simulink model "linearized_wave_model"  (R2020a)
settings: Solver=FixedStepAuto  StartTime=0.0  StopTime=2000  RelTol=1e-3
values from neighbouring files (symbols this model uses):
  east_drift_limit = 2    [wave_parameters.mat]
  k_down = 1.3    [wave_parameters.mat]
  k_east = 2    [wave_parameters.mat]
  k_north = 2    [wave_parameters.mat]
  k_pitch = 3    [wave_parameters.mat]
  k_roll = 3    [wave_parameters.mat]
  k_yaw = 3    [wave_parameters.mat]
  north_drift_limit = 2    [wave_parameters.mat]
  peak_frequency = 0.8    [wave_parameters.mat]
  wave_height = 1    [wave_parameters.mat]
  yaw_drift_limit = 0.174532925199    [wave_parameters.mat]
libraries: simulink x9
settings Model: Creator=thomas.evang  LastModifiedBy=thomas.evang
settings RTWCC: Description=Generic Real-Time Target

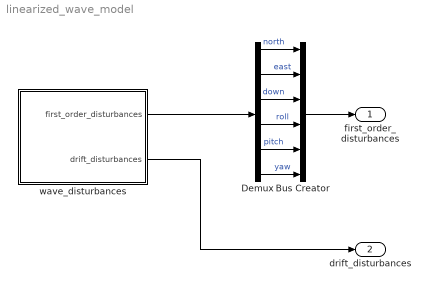
== system linearized_wave_model ==
  Bus Creator : BusCreator  Inputs=6  OutDataTypeStr=Bus: wave_disturbance
  Demux : Demux  Outputs=6
  wave_disturbances : Subsystem  mask{Hs=wave_height, w0=peak_frequency, k_north=k_north, k_east=k_east, k_down=k_down, k_roll=k_roll, k_pitch=k_pitch, k_yaw=k_yaw}
      mask prompts: Hs "Significant Wave Height"; w0 "Peak Frequency"; k_north "North Coefficient"; k_east "East Coefficient"; k_down "Down Coefficient"; k_roll "Roll Coefficient"; k_pitch "Pitch Coefficient"; k_yaw "Yaw Coefficient"
  first_order_disturbances : Outport  OutDataTypeStr=Bus: wave_disturbance
  drift_disturbances : Outport  Port=2  OutDataTypeStr=Bus: position_6dof
  wires:
  wave_disturbances/1(first_order_disturbances) -> Demux/1
  Demux/2 -> Bus Creator/2  "east"
  Demux/1 -> Bus Creator/1  "north"
  Demux/3 -> Bus Creator/3  "down"
  Demux/4 -> Bus Creator/4  "roll"
  Demux/5 -> Bus Creator/5  "pitch"
  Demux/6 -> Bus Creator/6  "yaw"
  Bus Creator/1 -> first_order_disturbances/1
  wave_disturbances/2(drift_disturbances) -> drift_disturbances/1

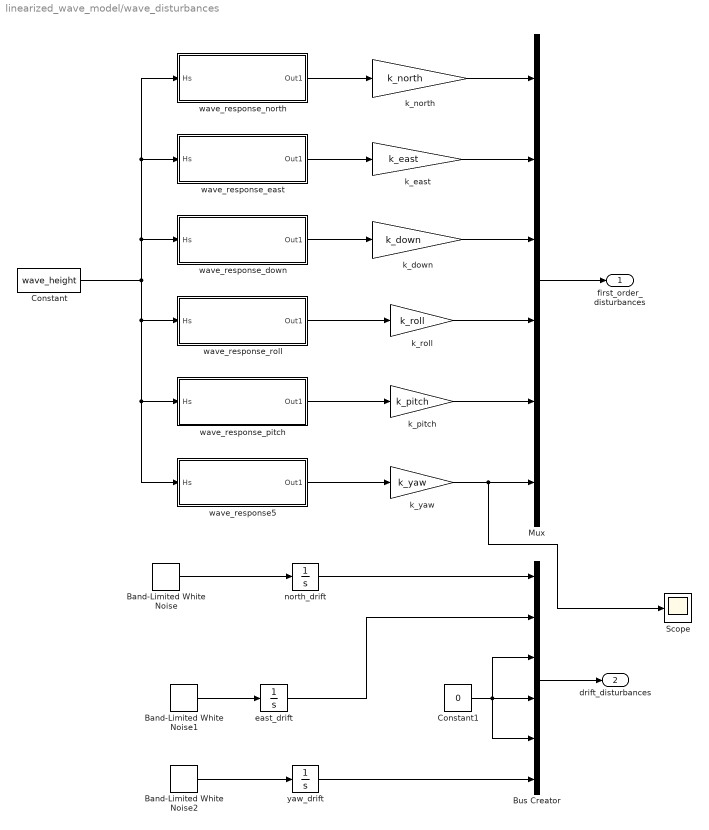
== system linearized_wave_model/wave_disturbances ==
  Band-Limited White Noise : simulink/Sources/Band-Limited White Noise  Cov=[0.005]  Ts=0.1  seed=[23341]
  Band-Limited White Noise1 : simulink/Sources/Band-Limited White Noise  Cov=[0.005]  Ts=0.1  seed=[23341]
  Band-Limited White Noise2 : simulink/Sources/Band-Limited White Noise  Cov=[0.005]  Ts=0.1  seed=[23341]
  Bus Creator : BusCreator  Inputs=6  OutDataTypeStr=Bus: position_6dof
      settings: InheritFromInputs=off
  Constant : Constant  Value=wave_height
  Constant1 : Constant  Value=0
  Mux : Mux  Inputs=6
  Scope : Scope
  east_drift : Integrator  LimitOutput=on  UpperSaturationLimit=east_drift_limit  LowerSaturationLimit=-east_drift_limit
  k_down : Gain  Gain=k_down
  k_east : Gain  Gain=k_east
  k_north : Gain  Gain=k_north
  k_pitch : Gain  Gain=k_pitch
  k_roll : Gain  Gain=k_roll
  k_yaw : Gain  Gain=k_yaw
  north_drift : Integrator  LimitOutput=on  UpperSaturationLimit=north_drift_limit  LowerSaturationLimit=-north_drift_limit
  wave_response5 : Subsystem  mask{w0=peak_frequency}
      mask prompts: w0 "Peak Frequency"
  wave_response_down : Subsystem  mask{w0=peak_frequency}
      mask prompts: w0 "Peak Frequency"
  wave_response_east : Subsystem  mask{w0=peak_frequency}
      mask prompts: w0 "Peak Frequency"
  wave_response_north : Subsystem  mask{w0=peak_frequency}
      mask prompts: w0 "Peak Frequency"
  wave_response_pitch : Subsystem  mask{w0=peak_frequency}
      mask prompts: w0 "Peak Frequency"
  wave_response_roll : Subsystem  mask{w0=peak_frequency}
      mask prompts: w0 "Peak Frequency"
  yaw_drift : Integrator  LimitOutput=on  UpperSaturationLimit=yaw_drift_limit  LowerSaturationLimit=-yaw_drift_limit
  first_order_disturbances : Outport
  drift_disturbances : Outport  Port=2
  wires:
  k_pitch/1 -> Mux/5
  k_yaw/1 -> Scope/1, Mux/6
  Mux/1 -> first_order_disturbances/1
  k_north/1 -> Mux/1
  k_down/1 -> Mux/3
  k_east/1 -> Mux/2
  k_roll/1 -> Mux/4
  Constant/1 -> wave_response_north/1(Hs), wave_response_east/1(Hs), wave_response_down/1(Hs), wave_response_roll/1(Hs), wave_response_pitch/1(Hs), wave_response5/1(Hs)
  wave_response_north/1(Out1) -> k_north/1
  wave_response_east/1(Out1) -> k_east/1
  wave_response_down/1(Out1) -> k_down/1
  wave_response_roll/1(Out1) -> k_roll/1
  wave_response_pitch/1(Out1) -> k_pitch/1
  wave_response5/1(Out1) -> k_yaw/1
  north_drift/1 -> Bus Creator/1
  east_drift/1 -> Bus Creator/2
  Bus Creator/1 -> drift_disturbances/1
  yaw_drift/1 -> Bus Creator/6
  Constant1/1 -> Bus Creator/5, Bus Creator/4, Bus Creator/3
  Band-Limited White Noise1/1 -> east_drift/1
  Band-Limited White Noise2/1 -> yaw_drift/1
  Band-Limited White Noise/1 -> north_drift/1

== system linearized_wave_model/wave_disturbances/wave_response5 ==
  Hs : Inport
  Band-Limited White Noise : simulink/Sources/Band-Limited White Noise  Cov=0.5  Ts=0.1  seed=[23341]
  C : Gain  Gain=[0 1]  Multiplication=Matrix(K*u)
  Gain : Gain  Gain="[0 1; -peak_frequency^2  -2*0.1017*peak_frequency]"  Multiplication=Matrix(K*u)
  Gain1 : Gain  Gain=[0; 1]  Multiplication=Matrix(K*u)
  Integrator : Integrator  InitialCondition=[0; 0]
  K_w : Subsystem  mask{lambda=0.1017, w0=w0}
      mask prompts: w0 "Peak Frequency"
  MatrixMultiply : Product
  Sum : Sum  Inputs=|++
  Out1 : Outport
  wires:
  Band-Limited White Noise/1 -> Gain1/1
  MatrixMultiply/1 -> Sum/1
  Gain/1 -> Sum/2
  Sum/1 -> Integrator/1
  Gain1/1 -> MatrixMultiply/2
  K_w/1(K_w) -> MatrixMultiply/1
  Hs/1 -> K_w/1(Hs)
  Integrator/1 -> Gain/1, C/1
  C/1 -> Out1/1

== system linearized_wave_model/wave_disturbances/wave_response_down ==
  Hs : Inport
  Band-Limited White Noise : simulink/Sources/Band-Limited White Noise  Cov=1  Ts=0.1  seed=[23341]
  C : Gain  Gain=[0 1]  Multiplication=Matrix(K*u)
  Gain : Gain  Gain="[0 1; -peak_frequency^2  -2*0.1017*peak_frequency]"  Multiplication=Matrix(K*u)
  Gain1 : Gain  Gain=[0; 1]  Multiplication=Matrix(K*u)
  Integrator : Integrator  InitialCondition=[0; 0]
  K_w : Subsystem  mask{lambda=0.1017, w0=w0}
      mask prompts: w0 "Peak Frequency"
  MatrixMultiply : Product
  Sum : Sum  Inputs=|++
  Out1 : Outport
  wires:
  Integrator/1 -> C/1, Gain/1
  Hs/1 -> K_w/1(Hs)
  K_w/1(K_w) -> MatrixMultiply/1
  Gain1/1 -> MatrixMultiply/2
  Sum/1 -> Integrator/1
  Gain/1 -> Sum/2
  MatrixMultiply/1 -> Sum/1
  Band-Limited White Noise/1 -> Gain1/1
  C/1 -> Out1/1

== system linearized_wave_model/wave_disturbances/wave_response_east ==
  Hs : Inport
  Band-Limited White Noise : simulink/Sources/Band-Limited White Noise  Cov=1  Ts=0.1  seed=[23341]
  C : Gain  Gain=[0 1]  Multiplication=Matrix(K*u)
  Gain : Gain  Gain="[0 1; -peak_frequency^2  -2*0.1017*peak_frequency]"  Multiplication=Matrix(K*u)
  Gain1 : Gain  Gain=[0; 1]  Multiplication=Matrix(K*u)
  Integrator : Integrator  InitialCondition=[0; 0]
  K_w : Subsystem  mask{lambda=0.1017, w0=w0}
      mask prompts: w0 "Peak Frequency"
  MatrixMultiply : Product
  Sum : Sum  Inputs=|++
  Out1 : Outport
  wires:
  Band-Limited White Noise/1 -> Gain1/1
  MatrixMultiply/1 -> Sum/1
  Gain/1 -> Sum/2
  Sum/1 -> Integrator/1
  Gain1/1 -> MatrixMultiply/2
  K_w/1(K_w) -> MatrixMultiply/1
  Hs/1 -> K_w/1(Hs)
  Integrator/1 -> Gain/1, C/1
  C/1 -> Out1/1

== system linearized_wave_model/wave_disturbances/wave_response_north ==
  Hs : Inport
  Band-Limited White Noise : simulink/Sources/Band-Limited White Noise  Cov=1  Ts=0.1  seed=[23341]
  C : Gain  Gain=[0 1]  Multiplication=Matrix(K*u)
  Gain : Gain  Gain="[0 1; -peak_frequency^2  -2*0.1017*peak_frequency]"  Multiplication=Matrix(K*u)
  Gain1 : Gain  Gain=[0; 1]  Multiplication=Matrix(K*u)
  Integrator : Integrator  InitialCondition=[0; 0]
  K_w : Subsystem  mask{lambda=0.1017, w0=w0}
      mask prompts: w0 "Peak Frequency"
  MatrixMultiply : Product
  Sum : Sum  Inputs=|++
  Out1 : Outport
  wires:
  Integrator/1 -> C/1, Gain/1
  Hs/1 -> K_w/1(Hs)
  K_w/1(K_w) -> MatrixMultiply/1
  Gain1/1 -> MatrixMultiply/2
  Sum/1 -> Integrator/1
  Gain/1 -> Sum/2
  MatrixMultiply/1 -> Sum/1
  Band-Limited White Noise/1 -> Gain1/1
  C/1 -> Out1/1

== system linearized_wave_model/wave_disturbances/wave_response_pitch ==
  Hs : Inport
  Band-Limited White Noise : simulink/Sources/Band-Limited White Noise  Cov=1  Ts=0.1  seed=[23341]
  C : Gain  Gain=[0 1]  Multiplication=Matrix(K*u)
  Gain : Gain  Gain="[0 1; -peak_frequency^2  -2*0.1017*peak_frequency]"  Multiplication=Matrix(K*u)
  Gain1 : Gain  Gain=[0; 1]  Multiplication=Matrix(K*u)
  Integrator : Integrator  InitialCondition=[0; 0]
  K_w : Subsystem  mask{lambda=0.1017, w0=w0}
      mask prompts: w0 "Peak Frequency"
  MatrixMultiply : Product
  Sum : Sum  Inputs=|++
  Out1 : Outport
  wires:
  Integrator/1 -> C/1, Gain/1
  Hs/1 -> K_w/1(Hs)
  K_w/1(K_w) -> MatrixMultiply/1
  Gain1/1 -> MatrixMultiply/2
  Sum/1 -> Integrator/1
  Gain/1 -> Sum/2
  MatrixMultiply/1 -> Sum/1
  Band-Limited White Noise/1 -> Gain1/1
  C/1 -> Out1/1

== system linearized_wave_model/wave_disturbances/wave_response_roll ==
  Hs : Inport
  Band-Limited White Noise : simulink/Sources/Band-Limited White Noise  Cov=1  Ts=0.1  seed=[23341]
  C : Gain  Gain=[0 1]  Multiplication=Matrix(K*u)
  Gain : Gain  Gain="[0 1; -peak_frequency^2  -2*0.1017*peak_frequency]"  Multiplication=Matrix(K*u)
  Gain1 : Gain  Gain=[0; 1]  Multiplication=Matrix(K*u)
  Integrator : Integrator  InitialCondition=[0; 0]
  K_w : Subsystem  mask{lambda=0.1017, w0=w0}
      mask prompts: w0 "Peak Frequency"
  MatrixMultiply : Product
  Sum : Sum  Inputs=|++
  Out1 : Outport
  wires:
  Band-Limited White Noise/1 -> Gain1/1
  MatrixMultiply/1 -> Sum/1
  Gain/1 -> Sum/2
  Sum/1 -> Integrator/1
  Gain1/1 -> MatrixMultiply/2
  K_w/1(K_w) -> MatrixMultiply/1
  Hs/1 -> K_w/1(Hs)
  Integrator/1 -> Gain/1, C/1
  C/1 -> Out1/1

== system linearized_wave_model/wave_disturbances/wave_response5/K_w ==
  Hs : Inport
  Gain : Gain  Gain=2*lambda*w0
  Sigma : Subsystem
  K_w : Outport
  wires:
  Hs/1 -> Sigma/1(Hs)
  Sigma/1(sigma) -> Gain/1
  Gain/1 -> K_w/1

== system linearized_wave_model/wave_disturbances/wave_response_down/K_w ==
  Hs : Inport
  Gain : Gain  Gain=2*lambda*w0
  Sigma : Subsystem
  K_w : Outport
  wires:
  Gain/1 -> K_w/1
  Sigma/1(sigma) -> Gain/1
  Hs/1 -> Sigma/1(Hs)

== system linearized_wave_model/wave_disturbances/wave_response_east/K_w ==
  Hs : Inport
  Gain : Gain  Gain=2*lambda*w0
  Sigma : Subsystem
  K_w : Outport
  wires:
  Hs/1 -> Sigma/1(Hs)
  Sigma/1(sigma) -> Gain/1
  Gain/1 -> K_w/1

== system linearized_wave_model/wave_disturbances/wave_response_north/K_w ==
  Hs : Inport
  Gain : Gain  Gain=2*lambda*w0
  Sigma : Subsystem
  K_w : Outport
  wires:
  Gain/1 -> K_w/1
  Sigma/1(sigma) -> Gain/1
  Hs/1 -> Sigma/1(Hs)

== system linearized_wave_model/wave_disturbances/wave_response_pitch/K_w ==
  Hs : Inport
  Gain : Gain  Gain=2*lambda*w0
  Sigma : Subsystem
  K_w : Outport
  wires:
  Gain/1 -> K_w/1
  Sigma/1(sigma) -> Gain/1
  Hs/1 -> Sigma/1(Hs)

== system linearized_wave_model/wave_disturbances/wave_response_roll/K_w ==
  Hs : Inport
  Gain : Gain  Gain=2*lambda*w0
  Sigma : Subsystem
  K_w : Outport
  wires:
  Hs/1 -> Sigma/1(Hs)
  Sigma/1(sigma) -> Gain/1
  Gain/1 -> K_w/1

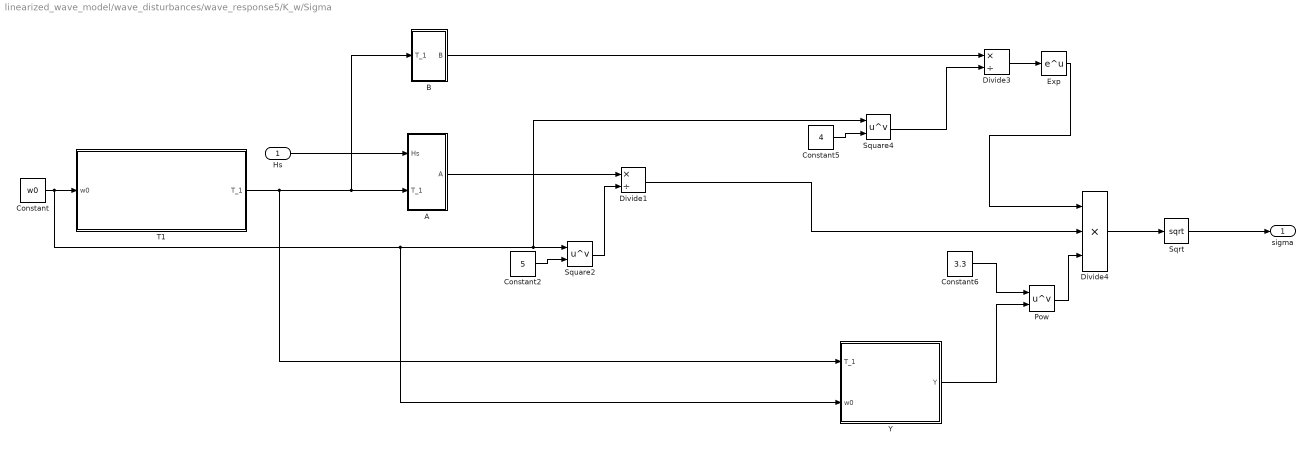
== system linearized_wave_model/wave_disturbances/wave_response5/K_w/Sigma ==
  Hs : Inport
  A : Subsystem
  B : Subsystem
  Constant : Constant  Value=w0
  Constant2 : Constant  Value=5
  Constant5 : Constant  Value=4
  Constant6 : Constant  Value=3.3
  Divide1 : Product  Inputs=*/
  Divide3 : Product  Inputs=*/
  Divide4 : Product  Inputs=***
  Exp : Math  SaturateOnIntegerOverflow=on
  Pow : Math  Operator=pow  RndMeth=Zero  SaturateOnIntegerOverflow=on
  Sqrt : Sqrt  SaturateOnIntegerOverflow=on
  Square2 : Math  Operator=pow  SaturateOnIntegerOverflow=on
  Square4 : Math  Operator=pow  SaturateOnIntegerOverflow=on
  T1 : Subsystem
  Y : Subsystem
  sigma : Outport
  wires:
  B/1(B) -> Divide3/1
  A/1(A) -> Divide1/1
  Hs/1 -> A/1(Hs)
  Sqrt/1 -> sigma/1
  Divide4/1 -> Sqrt/1
  Pow/1 -> Divide4/3
  Y/1(Y) -> Pow/2
  Constant6/1 -> Pow/1
  Exp/1 -> Divide4/1
  Divide3/1 -> Exp/1
  Square4/1 -> Divide3/2
  Constant5/1 -> Square4/2
  Divide1/1 -> Divide4/2
  Square2/1 -> Divide1/2
  Constant2/1 -> Square2/2
  T1/1(T_1) -> A/2(T_1), B/1(T_1), Y/1(T_1)
  Constant/1 -> T1/1(w0), Square2/1, Square4/1, Y/2(w0)

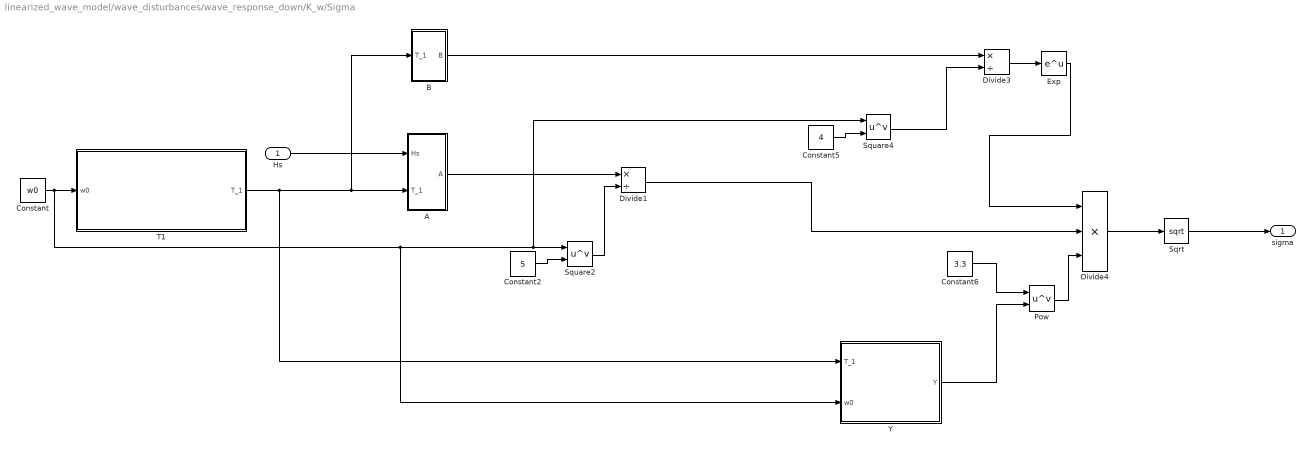
== system linearized_wave_model/wave_disturbances/wave_response_down/K_w/Sigma ==
  Hs : Inport
  A : Subsystem
  B : Subsystem
  Constant : Constant  Value=w0
  Constant2 : Constant  Value=5
  Constant5 : Constant  Value=4
  Constant6 : Constant  Value=3.3
  Divide1 : Product  Inputs=*/
  Divide3 : Product  Inputs=*/
  Divide4 : Product  Inputs=***
  Exp : Math  SaturateOnIntegerOverflow=on
  Pow : Math  Operator=pow  RndMeth=Zero  SaturateOnIntegerOverflow=on
  Sqrt : Sqrt  SaturateOnIntegerOverflow=on
  Square2 : Math  Operator=pow  SaturateOnIntegerOverflow=on
  Square4 : Math  Operator=pow  SaturateOnIntegerOverflow=on
  T1 : Subsystem
  Y : Subsystem
  sigma : Outport
  wires:
  Constant/1 -> Y/2(w0), Square4/1, Square2/1, T1/1(w0)
  T1/1(T_1) -> Y/1(T_1), B/1(T_1), A/2(T_1)
  Constant2/1 -> Square2/2
  Square2/1 -> Divide1/2
  Divide1/1 -> Divide4/2
  Constant5/1 -> Square4/2
  Square4/1 -> Divide3/2
  Divide3/1 -> Exp/1
  Exp/1 -> Divide4/1
  Constant6/1 -> Pow/1
  Y/1(Y) -> Pow/2
  Pow/1 -> Divide4/3
  Divide4/1 -> Sqrt/1
  Sqrt/1 -> sigma/1
  Hs/1 -> A/1(Hs)
  A/1(A) -> Divide1/1
  B/1(B) -> Divide3/1

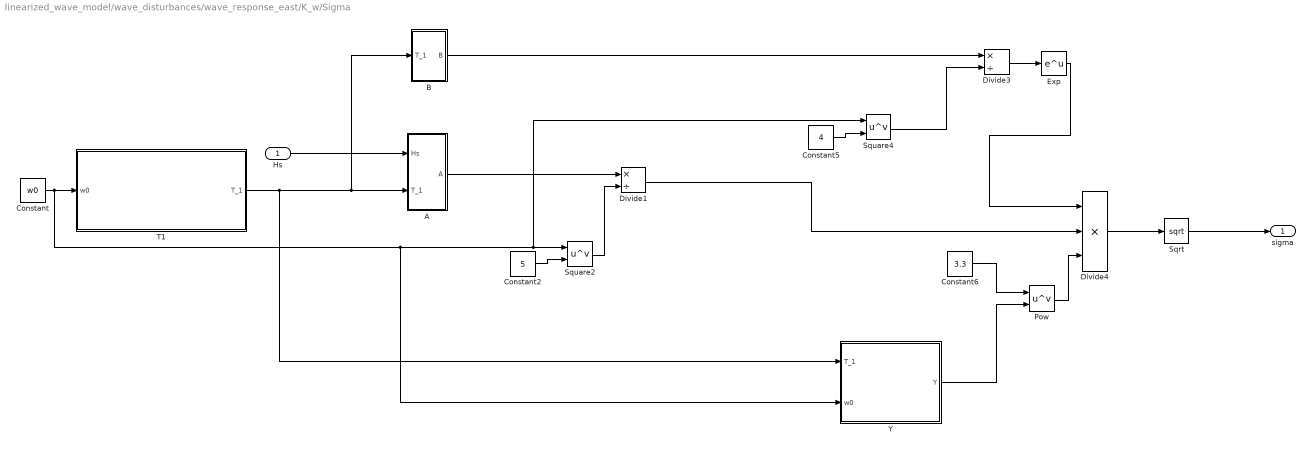
== system linearized_wave_model/wave_disturbances/wave_response_east/K_w/Sigma ==
  Hs : Inport
  A : Subsystem
  B : Subsystem
  Constant : Constant  Value=w0
  Constant2 : Constant  Value=5
  Constant5 : Constant  Value=4
  Constant6 : Constant  Value=3.3
  Divide1 : Product  Inputs=*/
  Divide3 : Product  Inputs=*/
  Divide4 : Product  Inputs=***
  Exp : Math  SaturateOnIntegerOverflow=on
  Pow : Math  Operator=pow  RndMeth=Zero  SaturateOnIntegerOverflow=on
  Sqrt : Sqrt  SaturateOnIntegerOverflow=on
  Square2 : Math  Operator=pow  SaturateOnIntegerOverflow=on
  Square4 : Math  Operator=pow  SaturateOnIntegerOverflow=on
  T1 : Subsystem
  Y : Subsystem
  sigma : Outport
  wires:
  B/1(B) -> Divide3/1
  A/1(A) -> Divide1/1
  Hs/1 -> A/1(Hs)
  Sqrt/1 -> sigma/1
  Divide4/1 -> Sqrt/1
  Pow/1 -> Divide4/3
  Y/1(Y) -> Pow/2
  Constant6/1 -> Pow/1
  Exp/1 -> Divide4/1
  Divide3/1 -> Exp/1
  Square4/1 -> Divide3/2
  Constant5/1 -> Square4/2
  Divide1/1 -> Divide4/2
  Square2/1 -> Divide1/2
  Constant2/1 -> Square2/2
  T1/1(T_1) -> A/2(T_1), B/1(T_1), Y/1(T_1)
  Constant/1 -> T1/1(w0), Square2/1, Square4/1, Y/2(w0)

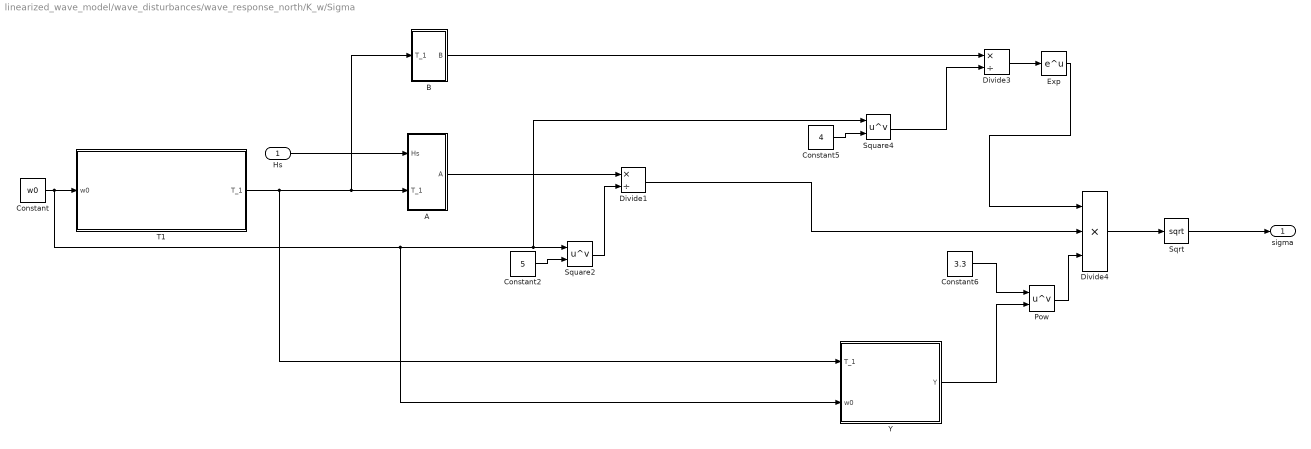
== system linearized_wave_model/wave_disturbances/wave_response_north/K_w/Sigma ==
  Hs : Inport
  A : Subsystem
  B : Subsystem
  Constant : Constant  Value=w0
  Constant2 : Constant  Value=5
  Constant5 : Constant  Value=4
  Constant6 : Constant  Value=3.3
  Divide1 : Product  Inputs=*/
  Divide3 : Product  Inputs=*/
  Divide4 : Product  Inputs=***
  Exp : Math  SaturateOnIntegerOverflow=on
  Pow : Math  Operator=pow  RndMeth=Zero  SaturateOnIntegerOverflow=on
  Sqrt : Sqrt  SaturateOnIntegerOverflow=on
  Square2 : Math  Operator=pow  SaturateOnIntegerOverflow=on
  Square4 : Math  Operator=pow  SaturateOnIntegerOverflow=on
  T1 : Subsystem
  Y : Subsystem
  sigma : Outport
  wires:
  Constant/1 -> Y/2(w0), Square4/1, Square2/1, T1/1(w0)
  T1/1(T_1) -> Y/1(T_1), B/1(T_1), A/2(T_1)
  Constant2/1 -> Square2/2
  Square2/1 -> Divide1/2
  Divide1/1 -> Divide4/2
  Constant5/1 -> Square4/2
  Square4/1 -> Divide3/2
  Divide3/1 -> Exp/1
  Exp/1 -> Divide4/1
  Constant6/1 -> Pow/1
  Y/1(Y) -> Pow/2
  Pow/1 -> Divide4/3
  Divide4/1 -> Sqrt/1
  Sqrt/1 -> sigma/1
  Hs/1 -> A/1(Hs)
  A/1(A) -> Divide1/1
  B/1(B) -> Divide3/1

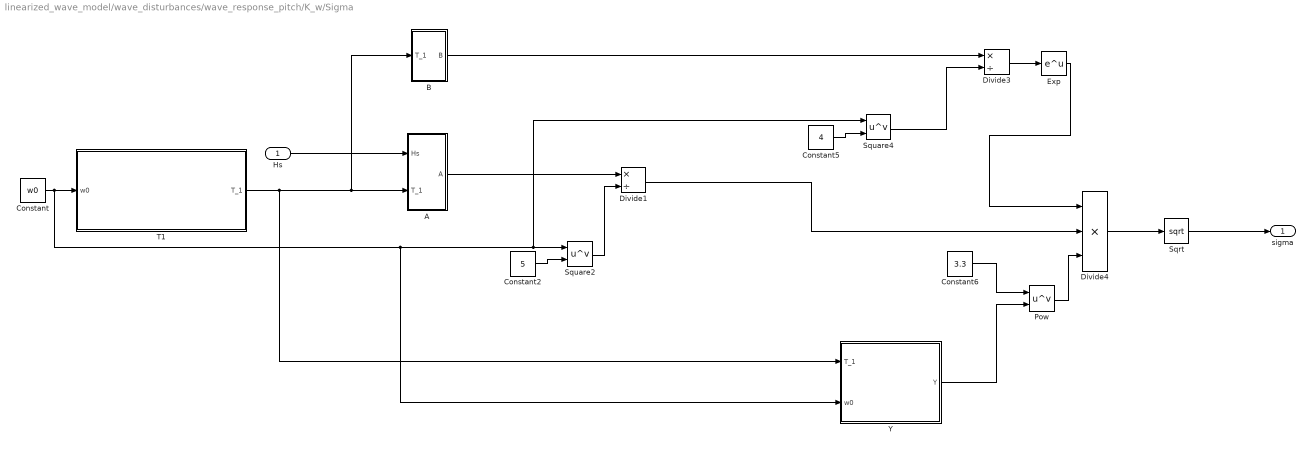
== system linearized_wave_model/wave_disturbances/wave_response_pitch/K_w/Sigma ==
  Hs : Inport
  A : Subsystem
  B : Subsystem
  Constant : Constant  Value=w0
  Constant2 : Constant  Value=5
  Constant5 : Constant  Value=4
  Constant6 : Constant  Value=3.3
  Divide1 : Product  Inputs=*/
  Divide3 : Product  Inputs=*/
  Divide4 : Product  Inputs=***
  Exp : Math  SaturateOnIntegerOverflow=on
  Pow : Math  Operator=pow  RndMeth=Zero  SaturateOnIntegerOverflow=on
  Sqrt : Sqrt  SaturateOnIntegerOverflow=on
  Square2 : Math  Operator=pow  SaturateOnIntegerOverflow=on
  Square4 : Math  Operator=pow  SaturateOnIntegerOverflow=on
  T1 : Subsystem
  Y : Subsystem
  sigma : Outport
  wires:
  Constant/1 -> Y/2(w0), Square4/1, Square2/1, T1/1(w0)
  T1/1(T_1) -> Y/1(T_1), B/1(T_1), A/2(T_1)
  Constant2/1 -> Square2/2
  Square2/1 -> Divide1/2
  Divide1/1 -> Divide4/2
  Constant5/1 -> Square4/2
  Square4/1 -> Divide3/2
  Divide3/1 -> Exp/1
  Exp/1 -> Divide4/1
  Constant6/1 -> Pow/1
  Y/1(Y) -> Pow/2
  Pow/1 -> Divide4/3
  Divide4/1 -> Sqrt/1
  Sqrt/1 -> sigma/1
  Hs/1 -> A/1(Hs)
  A/1(A) -> Divide1/1
  B/1(B) -> Divide3/1

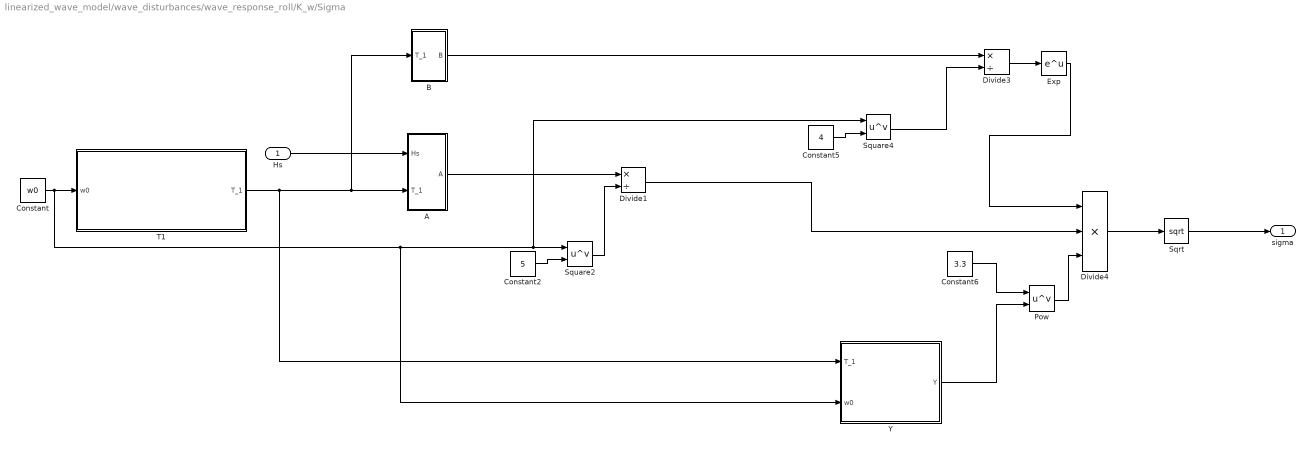
== system linearized_wave_model/wave_disturbances/wave_response_roll/K_w/Sigma ==
  Hs : Inport
  A : Subsystem
  B : Subsystem
  Constant : Constant  Value=w0
  Constant2 : Constant  Value=5
  Constant5 : Constant  Value=4
  Constant6 : Constant  Value=3.3
  Divide1 : Product  Inputs=*/
  Divide3 : Product  Inputs=*/
  Divide4 : Product  Inputs=***
  Exp : Math  SaturateOnIntegerOverflow=on
  Pow : Math  Operator=pow  RndMeth=Zero  SaturateOnIntegerOverflow=on
  Sqrt : Sqrt  SaturateOnIntegerOverflow=on
  Square2 : Math  Operator=pow  SaturateOnIntegerOverflow=on
  Square4 : Math  Operator=pow  SaturateOnIntegerOverflow=on
  T1 : Subsystem
  Y : Subsystem
  sigma : Outport
  wires:
  B/1(B) -> Divide3/1
  A/1(A) -> Divide1/1
  Hs/1 -> A/1(Hs)
  Sqrt/1 -> sigma/1
  Divide4/1 -> Sqrt/1
  Pow/1 -> Divide4/3
  Y/1(Y) -> Pow/2
  Constant6/1 -> Pow/1
  Exp/1 -> Divide4/1
  Divide3/1 -> Exp/1
  Square4/1 -> Divide3/2
  Constant5/1 -> Square4/2
  Divide1/1 -> Divide4/2
  Square2/1 -> Divide1/2
  Constant2/1 -> Square2/2
  T1/1(T_1) -> A/2(T_1), B/1(T_1), Y/1(T_1)
  Constant/1 -> T1/1(w0), Square2/1, Square4/1, Y/2(w0)

== system linearized_wave_model/wave_disturbances/wave_response5/K_w/Sigma/A ==
  Hs : Inport
  T_1 : Inport  Port=2
  Constant1 : Constant  Value=4
  Divide : Product  Inputs=*/
  Gain : Gain  Gain=155
  Square : Math  Operator=square  SaturateOnIntegerOverflow=on
  Square1 : Math  Operator=pow  SaturateOnIntegerOverflow=on
  A : Outport
  wires:
  T_1/1 -> Square1/1
  Divide/1 -> A/1
  Hs/1 -> Square/1
  Gain/1 -> Divide/1
  Constant1/1 -> Square1/2
  Square1/1 -> Divide/2
  Square/1 -> Gain/1

== system linearized_wave_model/wave_disturbances/wave_response5/K_w/Sigma/B ==
  T_1 : Inport
  Constant3 : Constant  Value=4
  Constant4 : Constant  Value=-944
  Divide2 : Product  Inputs=*/
  Square3 : Math  Operator=pow  SaturateOnIntegerOverflow=on
  B : Outport
  wires:
  T_1/1 -> Square3/1
  Divide2/1 -> B/1
  Square3/1 -> Divide2/2
  Constant3/1 -> Square3/2
  Constant4/1 -> Divide2/1

== system linearized_wave_model/wave_disturbances/wave_response5/K_w/Sigma/T1 ==
  w0 : Inport
  Constant : Constant  Value=2*pi
  Divide : Product  Inputs=*/
  Gain : Gain  Gain=0.834
  T_1 : Outport
  wires:
  Gain/1 -> T_1/1
  Divide/1 -> Gain/1
  Constant/1 -> Divide/1
  w0/1 -> Divide/2

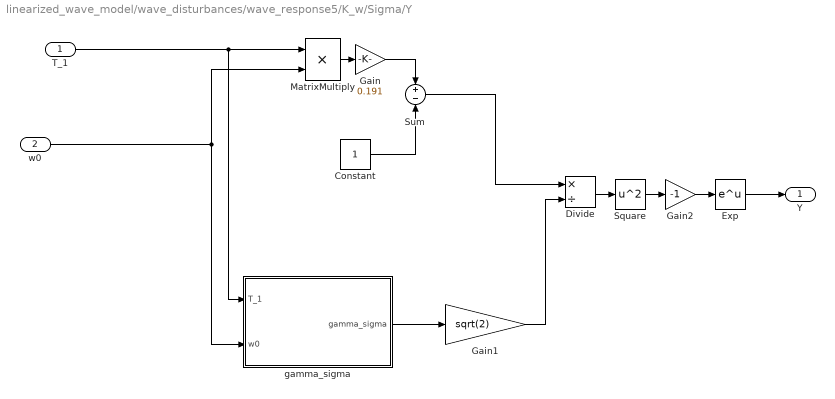
== system linearized_wave_model/wave_disturbances/wave_response5/K_w/Sigma/Y ==
  T_1 : Inport
  w0 : Inport  Port=2
  Constant : Constant
  Divide : Product  Inputs=*/
  Exp : Math  SaturateOnIntegerOverflow=on
  Gain : Gain  Gain=0.191
  Gain1 : Gain  Gain=sqrt(2)
  Gain2 : Gain  Gain=-1
  MatrixMultiply : Product
  Square : Math  Operator=square  SaturateOnIntegerOverflow=on
  Sum : Sum  Inputs=+|-
  gamma_sigma : Subsystem
  Y : Outport
  wires:
  Exp/1 -> Y/1
  Gain2/1 -> Exp/1
  Square/1 -> Gain2/1
  Divide/1 -> Square/1
  Gain1/1 -> Divide/2
  gamma_sigma/1(gamma_sigma) -> Gain1/1
  Sum/1 -> Divide/1
  Constant/1 -> Sum/2
  Gain/1 -> Sum/1
  MatrixMultiply/1 -> Gain/1
  w0/1 -> gamma_sigma/2(w0), MatrixMultiply/2
  T_1/1 -> gamma_sigma/1(T_1), MatrixMultiply/1

== system linearized_wave_model/wave_disturbances/wave_response_down/K_w/Sigma/A ==
  Hs : Inport
  T_1 : Inport  Port=2
  Constant1 : Constant  Value=4
  Divide : Product  Inputs=*/
  Gain : Gain  Gain=155
  Square : Math  Operator=square  SaturateOnIntegerOverflow=on
  Square1 : Math  Operator=pow  SaturateOnIntegerOverflow=on
  A : Outport
  wires:
  Square/1 -> Gain/1
  Square1/1 -> Divide/2
  Constant1/1 -> Square1/2
  Gain/1 -> Divide/1
  Hs/1 -> Square/1
  Divide/1 -> A/1
  T_1/1 -> Square1/1

== system linearized_wave_model/wave_disturbances/wave_response_down/K_w/Sigma/B ==
  T_1 : Inport
  Constant3 : Constant  Value=4
  Constant4 : Constant  Value=-944
  Divide2 : Product  Inputs=*/
  Square3 : Math  Operator=pow  SaturateOnIntegerOverflow=on
  B : Outport
  wires:
  Constant4/1 -> Divide2/1
  Constant3/1 -> Square3/2
  Square3/1 -> Divide2/2
  Divide2/1 -> B/1
  T_1/1 -> Square3/1

== system linearized_wave_model/wave_disturbances/wave_response_down/K_w/Sigma/T1 ==
  w0 : Inport
  Constant : Constant  Value=2*pi
  Divide : Product  Inputs=*/
  Gain : Gain  Gain=0.834
  T_1 : Outport
  wires:
  w0/1 -> Divide/2
  Constant/1 -> Divide/1
  Divide/1 -> Gain/1
  Gain/1 -> T_1/1

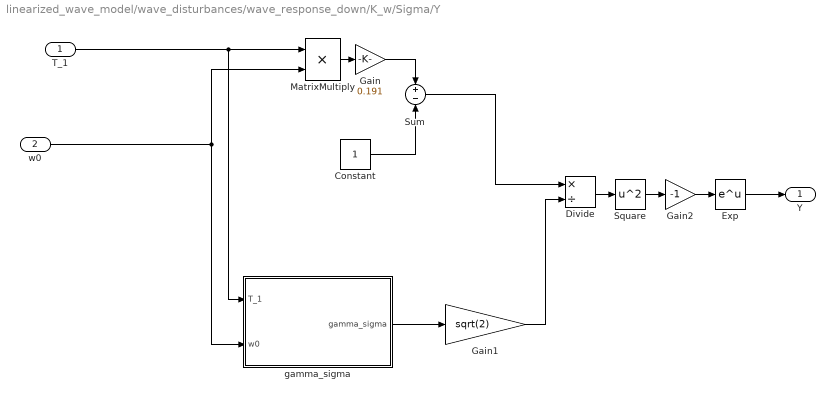
== system linearized_wave_model/wave_disturbances/wave_response_down/K_w/Sigma/Y ==
  T_1 : Inport
  w0 : Inport  Port=2
  Constant : Constant
  Divide : Product  Inputs=*/
  Exp : Math  SaturateOnIntegerOverflow=on
  Gain : Gain  Gain=0.191
  Gain1 : Gain  Gain=sqrt(2)
  Gain2 : Gain  Gain=-1
  MatrixMultiply : Product
  Square : Math  Operator=square  SaturateOnIntegerOverflow=on
  Sum : Sum  Inputs=+|-
  gamma_sigma : Subsystem
  Y : Outport
  wires:
  T_1/1 -> MatrixMultiply/1, gamma_sigma/1(T_1)
  w0/1 -> MatrixMultiply/2, gamma_sigma/2(w0)
  MatrixMultiply/1 -> Gain/1
  Gain/1 -> Sum/1
  Constant/1 -> Sum/2
  Sum/1 -> Divide/1
  gamma_sigma/1(gamma_sigma) -> Gain1/1
  Gain1/1 -> Divide/2
  Divide/1 -> Square/1
  Square/1 -> Gain2/1
  Gain2/1 -> Exp/1
  Exp/1 -> Y/1

== system linearized_wave_model/wave_disturbances/wave_response_east/K_w/Sigma/A ==
  Hs : Inport
  T_1 : Inport  Port=2
  Constant1 : Constant  Value=4
  Divide : Product  Inputs=*/
  Gain : Gain  Gain=155
  Square : Math  Operator=square  SaturateOnIntegerOverflow=on
  Square1 : Math  Operator=pow  SaturateOnIntegerOverflow=on
  A : Outport
  wires:
  T_1/1 -> Square1/1
  Divide/1 -> A/1
  Hs/1 -> Square/1
  Gain/1 -> Divide/1
  Constant1/1 -> Square1/2
  Square1/1 -> Divide/2
  Square/1 -> Gain/1

== system linearized_wave_model/wave_disturbances/wave_response_east/K_w/Sigma/B ==
  T_1 : Inport
  Constant3 : Constant  Value=4
  Constant4 : Constant  Value=-944
  Divide2 : Product  Inputs=*/
  Square3 : Math  Operator=pow  SaturateOnIntegerOverflow=on
  B : Outport
  wires:
  T_1/1 -> Square3/1
  Divide2/1 -> B/1
  Square3/1 -> Divide2/2
  Constant3/1 -> Square3/2
  Constant4/1 -> Divide2/1

== system linearized_wave_model/wave_disturbances/wave_response_east/K_w/Sigma/T1 ==
  w0 : Inport
  Constant : Constant  Value=2*pi
  Divide : Product  Inputs=*/
  Gain : Gain  Gain=0.834
  T_1 : Outport
  wires:
  Gain/1 -> T_1/1
  Divide/1 -> Gain/1
  Constant/1 -> Divide/1
  w0/1 -> Divide/2

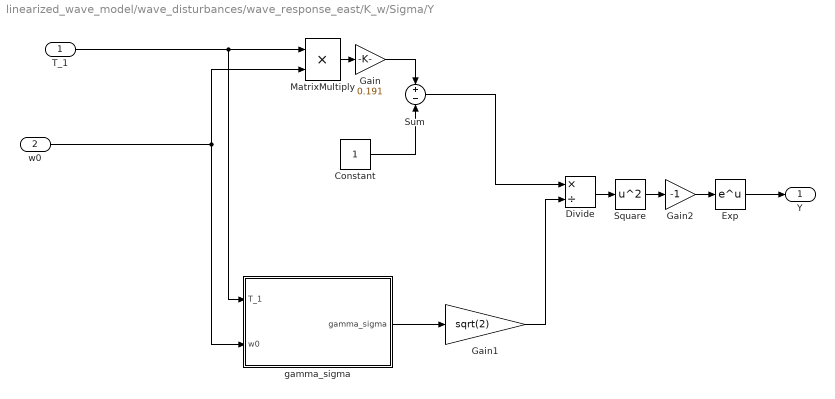
== system linearized_wave_model/wave_disturbances/wave_response_east/K_w/Sigma/Y ==
  T_1 : Inport
  w0 : Inport  Port=2
  Constant : Constant
  Divide : Product  Inputs=*/
  Exp : Math  SaturateOnIntegerOverflow=on
  Gain : Gain  Gain=0.191
  Gain1 : Gain  Gain=sqrt(2)
  Gain2 : Gain  Gain=-1
  MatrixMultiply : Product
  Square : Math  Operator=square  SaturateOnIntegerOverflow=on
  Sum : Sum  Inputs=+|-
  gamma_sigma : Subsystem
  Y : Outport
  wires:
  Exp/1 -> Y/1
  Gain2/1 -> Exp/1
  Square/1 -> Gain2/1
  Divide/1 -> Square/1
  Gain1/1 -> Divide/2
  gamma_sigma/1(gamma_sigma) -> Gain1/1
  Sum/1 -> Divide/1
  Constant/1 -> Sum/2
  Gain/1 -> Sum/1
  MatrixMultiply/1 -> Gain/1
  w0/1 -> gamma_sigma/2(w0), MatrixMultiply/2
  T_1/1 -> gamma_sigma/1(T_1), MatrixMultiply/1

== system linearized_wave_model/wave_disturbances/wave_response_north/K_w/Sigma/A ==
  Hs : Inport
  T_1 : Inport  Port=2
  Constant1 : Constant  Value=4
  Divide : Product  Inputs=*/
  Gain : Gain  Gain=155
  Square : Math  Operator=square  SaturateOnIntegerOverflow=on
  Square1 : Math  Operator=pow  SaturateOnIntegerOverflow=on
  A : Outport
  wires:
  Square/1 -> Gain/1
  Square1/1 -> Divide/2
  Constant1/1 -> Square1/2
  Gain/1 -> Divide/1
  Hs/1 -> Square/1
  Divide/1 -> A/1
  T_1/1 -> Square1/1

== system linearized_wave_model/wave_disturbances/wave_response_north/K_w/Sigma/B ==
  T_1 : Inport
  Constant3 : Constant  Value=4
  Constant4 : Constant  Value=-944
  Divide2 : Product  Inputs=*/
  Square3 : Math  Operator=pow  SaturateOnIntegerOverflow=on
  B : Outport
  wires:
  Constant4/1 -> Divide2/1
  Constant3/1 -> Square3/2
  Square3/1 -> Divide2/2
  Divide2/1 -> B/1
  T_1/1 -> Square3/1

== system linearized_wave_model/wave_disturbances/wave_response_north/K_w/Sigma/T1 ==
  w0 : Inport
  Constant : Constant  Value=2*pi
  Divide : Product  Inputs=*/
  Gain : Gain  Gain=0.834
  T_1 : Outport
  wires:
  w0/1 -> Divide/2
  Constant/1 -> Divide/1
  Divide/1 -> Gain/1
  Gain/1 -> T_1/1

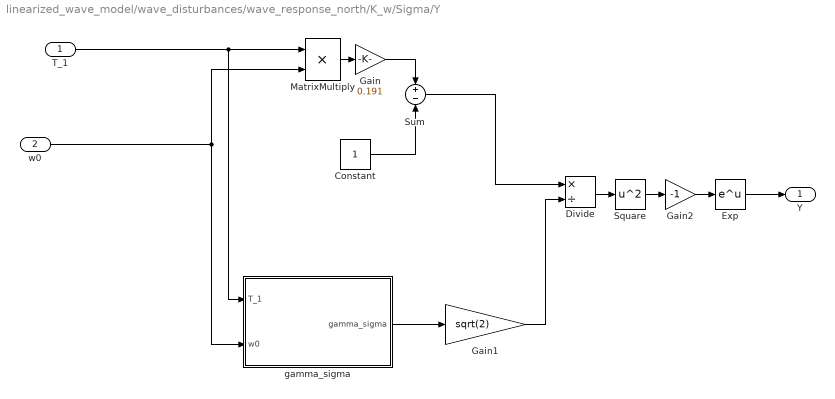
== system linearized_wave_model/wave_disturbances/wave_response_north/K_w/Sigma/Y ==
  T_1 : Inport
  w0 : Inport  Port=2
  Constant : Constant
  Divide : Product  Inputs=*/
  Exp : Math  SaturateOnIntegerOverflow=on
  Gain : Gain  Gain=0.191
  Gain1 : Gain  Gain=sqrt(2)
  Gain2 : Gain  Gain=-1
  MatrixMultiply : Product
  Square : Math  Operator=square  SaturateOnIntegerOverflow=on
  Sum : Sum  Inputs=+|-
  gamma_sigma : Subsystem
  Y : Outport
  wires:
  T_1/1 -> MatrixMultiply/1, gamma_sigma/1(T_1)
  w0/1 -> MatrixMultiply/2, gamma_sigma/2(w0)
  MatrixMultiply/1 -> Gain/1
  Gain/1 -> Sum/1
  Constant/1 -> Sum/2
  Sum/1 -> Divide/1
  gamma_sigma/1(gamma_sigma) -> Gain1/1
  Gain1/1 -> Divide/2
  Divide/1 -> Square/1
  Square/1 -> Gain2/1
  Gain2/1 -> Exp/1
  Exp/1 -> Y/1

== system linearized_wave_model/wave_disturbances/wave_response_pitch/K_w/Sigma/A ==
  Hs : Inport
  T_1 : Inport  Port=2
  Constant1 : Constant  Value=4
  Divide : Product  Inputs=*/
  Gain : Gain  Gain=155
  Square : Math  Operator=square  SaturateOnIntegerOverflow=on
  Square1 : Math  Operator=pow  SaturateOnIntegerOverflow=on
  A : Outport
  wires:
  Square/1 -> Gain/1
  Square1/1 -> Divide/2
  Constant1/1 -> Square1/2
  Gain/1 -> Divide/1
  Hs/1 -> Square/1
  Divide/1 -> A/1
  T_1/1 -> Square1/1

== system linearized_wave_model/wave_disturbances/wave_response_pitch/K_w/Sigma/B ==
  T_1 : Inport
  Constant3 : Constant  Value=4
  Constant4 : Constant  Value=-944
  Divide2 : Product  Inputs=*/
  Square3 : Math  Operator=pow  SaturateOnIntegerOverflow=on
  B : Outport
  wires:
  Constant4/1 -> Divide2/1
  Constant3/1 -> Square3/2
  Square3/1 -> Divide2/2
  Divide2/1 -> B/1
  T_1/1 -> Square3/1

== system linearized_wave_model/wave_disturbances/wave_response_pitch/K_w/Sigma/T1 ==
  w0 : Inport
  Constant : Constant  Value=2*pi
  Divide : Product  Inputs=*/
  Gain : Gain  Gain=0.834
  T_1 : Outport
  wires:
  w0/1 -> Divide/2
  Constant/1 -> Divide/1
  Divide/1 -> Gain/1
  Gain/1 -> T_1/1

== system linearized_wave_model/wave_disturbances/wave_response_pitch/K_w/Sigma/Y ==
  T_1 : Inport
  w0 : Inport  Port=2
  Constant : Constant
  Divide : Product  Inputs=*/
  Exp : Math  SaturateOnIntegerOverflow=on
  Gain : Gain  Gain=0.191
  Gain1 : Gain  Gain=sqrt(2)
  Gain2 : Gain  Gain=-1
  MatrixMultiply : Product
  Square : Math  Operator=square  SaturateOnIntegerOverflow=on
  Sum : Sum  Inputs=+|-
  gamma_sigma : Subsystem
  Y : Outport
  wires:
  T_1/1 -> MatrixMultiply/1, gamma_sigma/1(T_1)
  w0/1 -> MatrixMultiply/2, gamma_sigma/2(w0)
  MatrixMultiply/1 -> Gain/1
  Gain/1 -> Sum/1
  Constant/1 -> Sum/2
  Sum/1 -> Divide/1
  gamma_sigma/1(gamma_sigma) -> Gain1/1
  Gain1/1 -> Divide/2
  Divide/1 -> Square/1
  Square/1 -> Gain2/1
  Gain2/1 -> Exp/1
  Exp/1 -> Y/1

== system linearized_wave_model/wave_disturbances/wave_response_roll/K_w/Sigma/A ==
  Hs : Inport
  T_1 : Inport  Port=2
  Constant1 : Constant  Value=4
  Divide : Product  Inputs=*/
  Gain : Gain  Gain=155
  Square : Math  Operator=square  SaturateOnIntegerOverflow=on
  Square1 : Math  Operator=pow  SaturateOnIntegerOverflow=on
  A : Outport
  wires:
  T_1/1 -> Square1/1
  Divide/1 -> A/1
  Hs/1 -> Square/1
  Gain/1 -> Divide/1
  Constant1/1 -> Square1/2
  Square1/1 -> Divide/2
  Square/1 -> Gain/1

== system linearized_wave_model/wave_disturbances/wave_response_roll/K_w/Sigma/B ==
  T_1 : Inport
  Constant3 : Constant  Value=4
  Constant4 : Constant  Value=-944
  Divide2 : Product  Inputs=*/
  Square3 : Math  Operator=pow  SaturateOnIntegerOverflow=on
  B : Outport
  wires:
  T_1/1 -> Square3/1
  Divide2/1 -> B/1
  Square3/1 -> Divide2/2
  Constant3/1 -> Square3/2
  Constant4/1 -> Divide2/1

== system linearized_wave_model/wave_disturbances/wave_response_roll/K_w/Sigma/T1 ==
  w0 : Inport
  Constant : Constant  Value=2*pi
  Divide : Product  Inputs=*/
  Gain : Gain  Gain=0.834
  T_1 : Outport
  wires:
  Gain/1 -> T_1/1
  Divide/1 -> Gain/1
  Constant/1 -> Divide/1
  w0/1 -> Divide/2

== system linearized_wave_model/wave_disturbances/wave_response_roll/K_w/Sigma/Y ==
  T_1 : Inport
  w0 : Inport  Port=2
  Constant : Constant
  Divide : Product  Inputs=*/
  Exp : Math  SaturateOnIntegerOverflow=on
  Gain : Gain  Gain=0.191
  Gain1 : Gain  Gain=sqrt(2)
  Gain2 : Gain  Gain=-1
  MatrixMultiply : Product
  Square : Math  Operator=square  SaturateOnIntegerOverflow=on
  Sum : Sum  Inputs=+|-
  gamma_sigma : Subsystem
  Y : Outport
  wires:
  Exp/1 -> Y/1
  Gain2/1 -> Exp/1
  Square/1 -> Gain2/1
  Divide/1 -> Square/1
  Gain1/1 -> Divide/2
  gamma_sigma/1(gamma_sigma) -> Gain1/1
  Sum/1 -> Divide/1
  Constant/1 -> Sum/2
  Gain/1 -> Sum/1
  MatrixMultiply/1 -> Gain/1
  w0/1 -> gamma_sigma/2(w0), MatrixMultiply/2
  T_1/1 -> gamma_sigma/1(T_1), MatrixMultiply/1

== system linearized_wave_model/wave_disturbances/wave_response5/K_w/Sigma/Y/gamma_sigma ==
  T_1 : Inport
  w0 : Inport  Port=2
  Constant : Constant  Value=0.09
  Constant1 : Constant  Value=0.07
  MatrixMultiply : Product
  Switch : Switch  Criteria=u2 > Threshold  Threshold=5.24
  gamma_sigma : Outport
  wires:
  Switch/1 -> gamma_sigma/1
  Constant1/1 -> Switch/3
  Constant/1 -> Switch/1
  MatrixMultiply/1 -> Switch/2
  w0/1 -> MatrixMultiply/2
  T_1/1 -> MatrixMultiply/1

== system linearized_wave_model/wave_disturbances/wave_response_down/K_w/Sigma/Y/gamma_sigma ==
  T_1 : Inport
  w0 : Inport  Port=2
  Constant : Constant  Value=0.09
  Constant1 : Constant  Value=0.07
  MatrixMultiply : Product
  Switch : Switch  Criteria=u2 > Threshold  Threshold=5.24
  gamma_sigma : Outport
  wires:
  T_1/1 -> MatrixMultiply/1
  w0/1 -> MatrixMultiply/2
  MatrixMultiply/1 -> Switch/2
  Constant/1 -> Switch/1
  Constant1/1 -> Switch/3
  Switch/1 -> gamma_sigma/1

== system linearized_wave_model/wave_disturbances/wave_response_east/K_w/Sigma/Y/gamma_sigma ==
  T_1 : Inport
  w0 : Inport  Port=2
  Constant : Constant  Value=0.09
  Constant1 : Constant  Value=0.07
  MatrixMultiply : Product
  Switch : Switch  Criteria=u2 > Threshold  Threshold=5.24
  gamma_sigma : Outport
  wires:
  Switch/1 -> gamma_sigma/1
  Constant1/1 -> Switch/3
  Constant/1 -> Switch/1
  MatrixMultiply/1 -> Switch/2
  w0/1 -> MatrixMultiply/2
  T_1/1 -> MatrixMultiply/1

== system linearized_wave_model/wave_disturbances/wave_response_north/K_w/Sigma/Y/gamma_sigma ==
  T_1 : Inport
  w0 : Inport  Port=2
  Constant : Constant  Value=0.09
  Constant1 : Constant  Value=0.07
  MatrixMultiply : Product
  Switch : Switch  Criteria=u2 > Threshold  Threshold=5.24
  gamma_sigma : Outport
  wires:
  T_1/1 -> MatrixMultiply/1
  w0/1 -> MatrixMultiply/2
  MatrixMultiply/1 -> Switch/2
  Constant/1 -> Switch/1
  Constant1/1 -> Switch/3
  Switch/1 -> gamma_sigma/1

== system linearized_wave_model/wave_disturbances/wave_response_pitch/K_w/Sigma/Y/gamma_sigma ==
  T_1 : Inport
  w0 : Inport  Port=2
  Constant : Constant  Value=0.09
  Constant1 : Constant  Value=0.07
  MatrixMultiply : Product
  Switch : Switch  Criteria=u2 > Threshold  Threshold=5.24
  gamma_sigma : Outport
  wires:
  T_1/1 -> MatrixMultiply/1
  w0/1 -> MatrixMultiply/2
  MatrixMultiply/1 -> Switch/2
  Constant/1 -> Switch/1
  Constant1/1 -> Switch/3
  Switch/1 -> gamma_sigma/1

== system linearized_wave_model/wave_disturbances/wave_response_roll/K_w/Sigma/Y/gamma_sigma ==
  T_1 : Inport
  w0 : Inport  Port=2
  Constant : Constant  Value=0.09
  Constant1 : Constant  Value=0.07
  MatrixMultiply : Product
  Switch : Switch  Criteria=u2 > Threshold  Threshold=5.24
  gamma_sigma : Outport
  wires:
  Switch/1 -> gamma_sigma/1
  Constant1/1 -> Switch/3
  Constant/1 -> Switch/1
  MatrixMultiply/1 -> Switch/2
  w0/1 -> MatrixMultiply/2
  T_1/1 -> MatrixMultiply/1
